simulink model "Sameed_Ex_1_4"  (R2020a)
settings: Solver=VariableStepAuto  StartTime=0.0  StopTime=100  RelTol=1e-3
values from neighbouring files (symbols this model uses):
  initial_psi = 0    [init.m]
  initial_x0 = 0    [init.m]
  initial_y0 = -0.1    [init.m]
  input_velocity = 10    [init.m]
  kd = -0.0238    [init.m]
  kp = -0.0235    [init.m]
  length_front = 2    [init.m]
  length_rare = 0    [init.m]
libraries: simulink x1
settings Model: Creator=Sameed Quais  LastModifiedBy=Sameed Quais

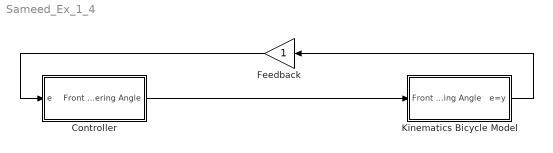
== system Sameed_Ex_1_4 ==
  Controller : Subsystem
  Feedback : Gain
  Kinematics Bicycle Model : Subsystem
  wires:
  Controller/1("Front Wheel Steering Angle ") -> Kinematics Bicycle Model/1("Front Wheel Steering Angle ")
  Kinematics Bicycle Model/1(e=y) -> Feedback/1
  Feedback/1 -> Controller/1(e)

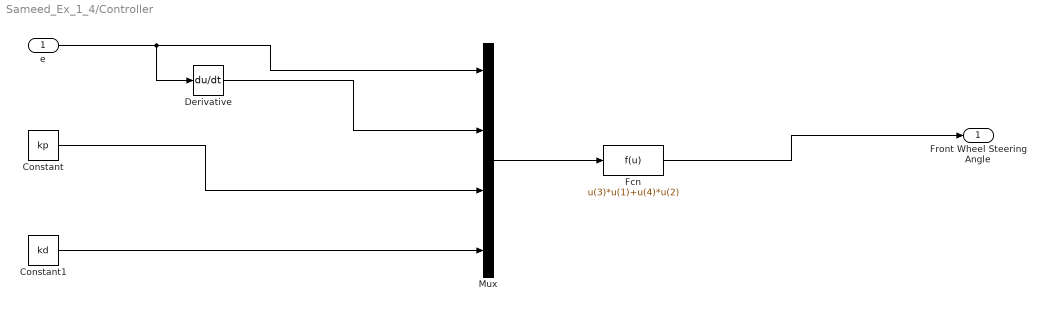
== system Sameed_Ex_1_4/Controller ==
  e : Inport
  Constant : Constant  Value=kp
  Constant1 : Constant  Value=kd
  Derivative : Derivative
  Fcn : Fcn  Expr=u(3)*u(1)+u(4)*u(2)
  Mux : Mux
  "Front Wheel Steering Angle " : Outport
  wires:
  e/1 -> Derivative/1, Mux/1
  Derivative/1 -> Mux/2
  Constant/1 -> Mux/3
  Constant1/1 -> Mux/4
  Mux/1 -> Fcn/1
  Fcn/1 -> "Front Wheel Steering Angle "/1

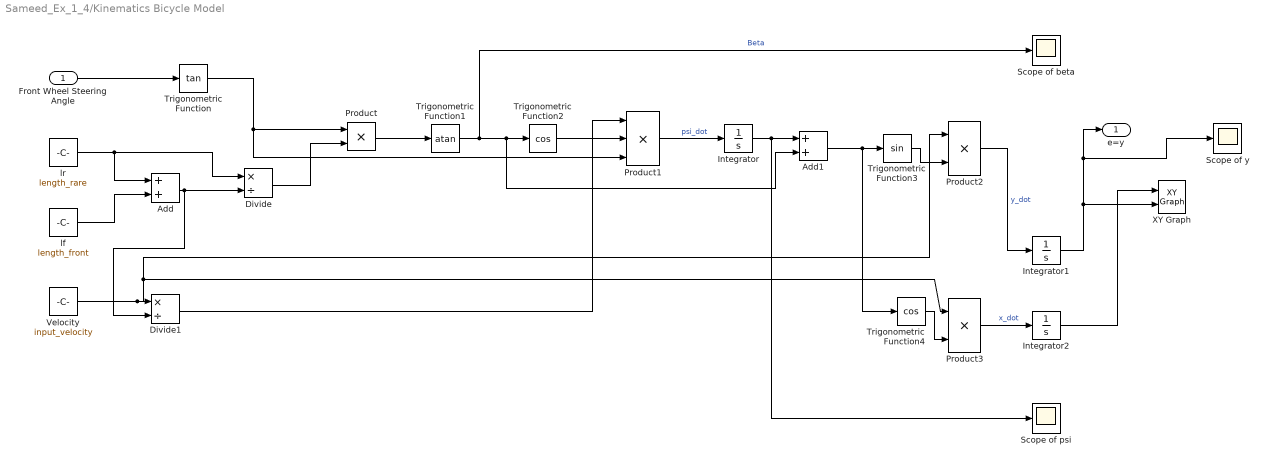
== system Sameed_Ex_1_4/Kinematics Bicycle Model ==
  "Front Wheel Steering Angle " : Inport
  Add : Sum
  Add1 : Sum
  Divide : Product  Inputs=*/
  Divide1 : Product  Inputs=*/
  Integrator : Integrator  InitialCondition=initial_psi
  Integrator1 : Integrator  InitialCondition=initial_y0
  Integrator2 : Integrator  InitialCondition=initial_x0
  Product : Product
  Product1 : Product  Inputs=3
  Product2 : Product
  Product3 : Product
  Scope of beta : Scope
  Scope of psi : Scope
  Scope of y : Scope
  Trigonometric Function : Trigonometry  Operator=tan
  Trigonometric Function1 : Trigonometry  Operator=atan
  Trigonometric Function2 : Trigonometry  Operator=cos
  Trigonometric Function3 : Trigonometry
  Trigonometric Function4 : Trigonometry  Operator=cos
  Velocity : Constant  Value=input_velocity
  XY Graph : simulink/Sinks/XY Graph  xmin=-1  xmax=100  ymin=-1  ymax=1  st=-1
  lf : Constant  Value=length_front
  lr : Constant  Value=length_rare
  e=y : Outport
  wires:
  "Front Wheel Steering Angle "/1 -> Trigonometric Function/1
  lr/1 -> Divide/1, Add/1
  lf/1 -> Add/2
  Trigonometric Function/1 -> Product1/3, Product/1
  Add/1 -> Divide1/2, Divide/2
  Divide/1 -> Product/2
  Product/1 -> Trigonometric Function1/1
  Trigonometric Function1/1 -> Scope of beta/1, Add1/2, Trigonometric Function2/1  "Beta"
  Trigonometric Function2/1 -> Product1/2
  Velocity/1 -> Product2/1, Product3/1, Divide1/1
  Divide1/1 -> Product1/1
  Product1/1 -> Integrator/1  "psi_dot"
  Integrator/1 -> Scope of psi/1, Add1/1
  Add1/1 -> Trigonometric Function4/1, Trigonometric Function3/1
  Trigonometric Function3/1 -> Product2/2
  Product2/1 -> Integrator1/1  "y_dot"
  Trigonometric Function4/1 -> Product3/2
  Product3/1 -> Integrator2/1  "x_dot"
  Integrator1/1 -> Scope of y/1, e=y/1, XY Graph/2
  Integrator2/1 -> XY Graph/1
